simulink model "ratio_esc_closed_loop"  (R2022b)
settings: Solver=FixedStepDiscrete  StartTime=0.0  StopTime=599.95000000000005  FixedStep=0.050000000000000003  RelTol=1e-3
model workspace (MAT data in the model file):
  noise_input = [0 0.05 0.1 0.15 0.2 0.25 0.3 0.35 0.4 0.45 0.5 0.55 ... (24000 elements, 12000x2)]
  optimum_input = [0 0.05 0.1 0.15 0.2 0.25 0.3 0.35 0.4 0.45 0.5 0.55 ... (24000 elements, 12000x2)]
  ratio_configuration : object (value not decoded)
libraries: simulink x1
(part 2 of 2)

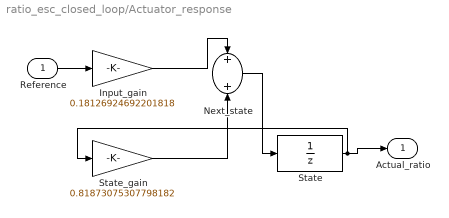
== system ratio_esc_closed_loop/Actuator_response ==
  Reference : Inport
  Input_gain : Gain  Gain=0.18126924692201818
  Next_state : Sum
  State : UnitDelay  InitialCondition=1.2  SampleTime=0.050000000000000003  HasFrameUpgradeWarning=on
  State_gain : Gain  Gain=0.81873075307798182
  Actual_ratio : Outport
  wires:
  Reference/1 -> Input_gain/1
  State/1 -> State_gain/1, Actual_ratio/1
  Input_gain/1 -> Next_state/1
  State_gain/1 -> Next_state/2
  Next_state/1 -> State/1

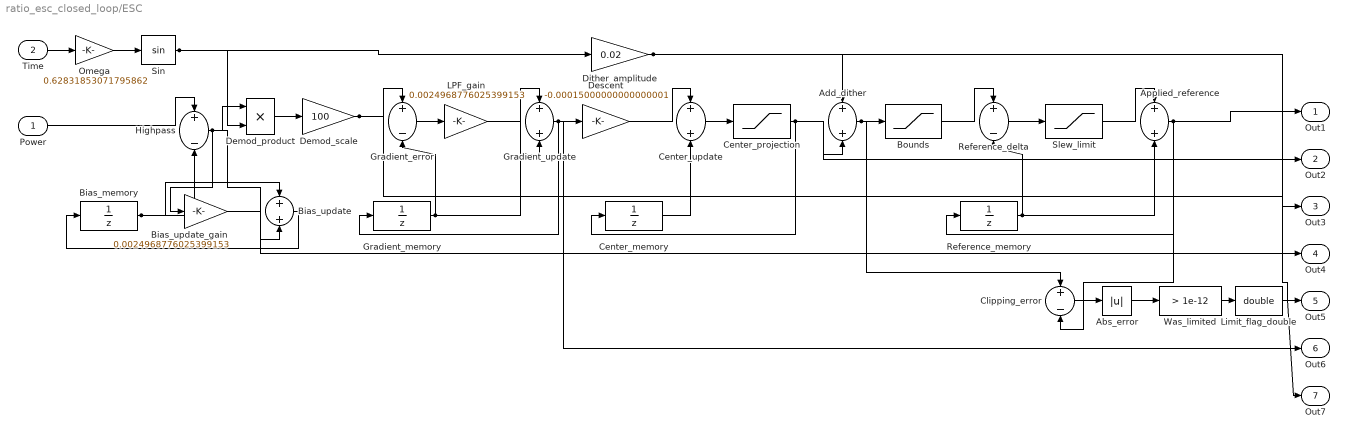
== system ratio_esc_closed_loop/ESC ==
  Power : Inport
  Time : Inport  Port=2
  Abs_error : Abs  SaturateOnIntegerOverflow=off
  Add_dither : Sum
  Applied_reference : Sum
  Bias_memory : UnitDelay  InitialCondition=1.3599999999999999  SampleTime=0.050000000000000003  HasFrameUpgradeWarning=on
  Bias_update : Sum
  Bias_update_gain : Gain  Gain=0.0024968776025399153
  Bounds : Saturate  UpperLimit=1.25  LowerLimit=0.75
  Center_memory : UnitDelay  InitialCondition=1.2  SampleTime=0.050000000000000003  HasFrameUpgradeWarning=on
  Center_projection : Saturate  UpperLimit=1.23  LowerLimit=0.77000000000000002
  Center_update : Sum
  Clipping_error : Sum  Inputs=+-
  Demod_product : Product
  Demod_scale : Gain  Gain=100
  Descent : Gain  Gain=-0.00015000000000000001
  Dither_amplitude : Gain  Gain=0.02
  Gradient_error : Sum  Inputs=+-
  Gradient_memory : UnitDelay  SampleTime=0.050000000000000003  HasFrameUpgradeWarning=on
  Gradient_update : Sum
  Highpass : Sum  Inputs=+-
  LPF_gain : Gain  Gain=0.0024968776025399153
  Limit_flag_double : DataTypeConversion  OutDataTypeStr=double  SaturateOnIntegerOverflow=off  RndMeth=Floor
  Omega : Gain  Gain=0.62831853071795862
  Reference_delta : Sum  Inputs=+-
  Reference_memory : UnitDelay  InitialCondition=1.2  SampleTime=0.050000000000000003  HasFrameUpgradeWarning=on
  Sin : Trigonometry
  Slew_limit : Saturate  UpperLimit=0.0025000000000000005  LowerLimit=-0.0025000000000000005
  Was_limited : simulink/Logic and Bit Operations/Compare To Constant  relop=>  const=1e-12  OutDataTypeStr=boolean
  Out1 : Outport
  Out2 : Outport  Port=2
  Out3 : Outport  Port=3
  Out4 : Outport  Port=4
  Out5 : Outport  Port=5
  Out6 : Outport  Port=6
  Out7 : Outport  Port=7
  wires:
  Time/1 -> Omega/1
  Omega/1 -> Sin/1
  Power/1 -> Highpass/1
  Bias_memory/1 -> Highpass/2, Bias_update/1
  Highpass/1 -> Bias_update_gain/1, Demod_product/1, Out4/1
  Bias_update_gain/1 -> Bias_update/2
  Bias_update/1 -> Bias_memory/1
  Sin/1 -> Demod_product/2, Dither_amplitude/1
  Demod_product/1 -> Demod_scale/1
  Demod_scale/1 -> Gradient_error/1, Out5/1
  Gradient_memory/1 -> Gradient_error/2, Gradient_update/1
  Gradient_error/1 -> LPF_gain/1
  LPF_gain/1 -> Gradient_update/2
  Gradient_update/1 -> Gradient_memory/1, Descent/1, Out6/1
  Descent/1 -> Center_update/1
  Center_memory/1 -> Center_update/2
  Center_update/1 -> Center_projection/1
  Center_projection/1 -> Center_memory/1, Add_dither/2, Out2/1
  Dither_amplitude/1 -> Add_dither/1, Out3/1
  Add_dither/1 -> Bounds/1, Clipping_error/1
  Bounds/1 -> Reference_delta/1
  Reference_memory/1 -> Reference_delta/2, Applied_reference/2
  Reference_delta/1 -> Slew_limit/1
  Slew_limit/1 -> Applied_reference/1
  Applied_reference/1 -> Reference_memory/1, Clipping_error/2, Out1/1
  Clipping_error/1 -> Abs_error/1
  Abs_error/1 -> Was_limited/1
  Was_limited/1 -> Limit_flag_double/1
  Limit_flag_double/1 -> Out7/1

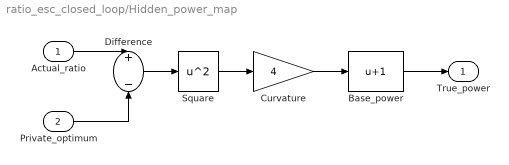
== system ratio_esc_closed_loop/Hidden_power_map ==
  Actual_ratio : Inport
  Private_optimum : Inport  Port=2
  Base_power : Bias  Bias=1  SaturateOnIntegerOverflow=off
  Curvature : Gain  Gain=4
  Difference : Sum  Inputs=+-
  Square : Math  Operator=square
  True_power : Outport
  wires:
  Actual_ratio/1 -> Difference/1
  Private_optimum/1 -> Difference/2
  Difference/1 -> Square/1
  Square/1 -> Curvature/1
  Curvature/1 -> Base_power/1
  Base_power/1 -> True_power/1

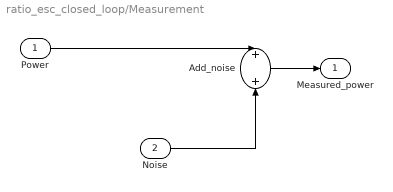
== system ratio_esc_closed_loop/Measurement ==
  Power : Inport
  Noise : Inport  Port=2
  Add_noise : Sum
  Measured_power : Outport
  wires:
  Power/1 -> Add_noise/1
  Noise/1 -> Add_noise/2
  Add_noise/1 -> Measured_power/1
